simulink model "mpcmodel"  (R2023a)
settings: Solver=VariableStepAuto  StartTime=0.0  StopTime=21  RelTol=1e-3
undefined symbols (not defined in the file): C_aug, C_l, C_m, disc_sys, init, min_sampling_time, mpc_kalman_gain, P, potentiometer_linearity_percent, Q, V_bar, wave_amplitude, wave_period, x1_bar, x2_bar
libraries: mpclib x1
settings Model: Creator=yunzh  LastModifiedBy=yunzh

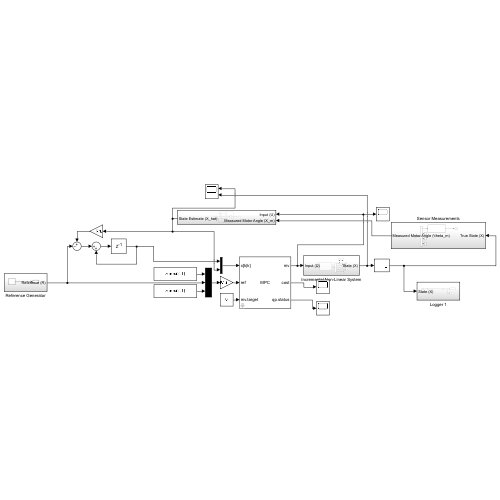
[thumbnail: Simulink's stored preview of the top-level diagram]
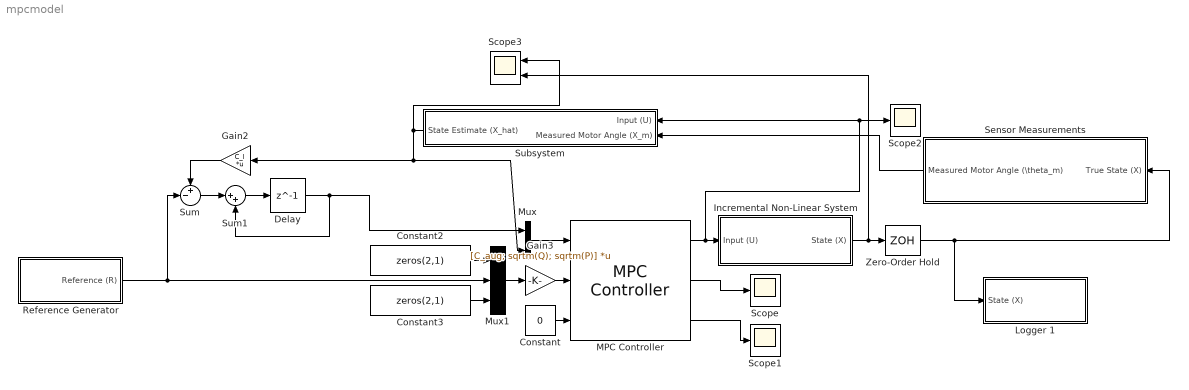
== system mpcmodel ==
  Constant : Constant  Value=0
  Constant2 : Constant  Value=zeros(2,1)
  Constant3 : Constant  Value=zeros(2,1)
  Delay : Delay  DelayLength=1  SampleTime=min_sampling_time
  Gain2 : Gain  Gain=C_l  Multiplication=Matrix(K*u)
  Gain3 : Gain  Gain=[C_aug; sqrtm(Q); sqrtm(P)]  Multiplication=Matrix(K*u)
  Incremental Non-Linear System : Subsystem
  Logger 1 : Subsystem
  MPC Controller : mpclib/MPC Controller  SCDEnableBlockLinearizationSpecification=on  mpcobj=mpc_obj  x0=mpc_initial_state  is_multiple=0  enable_value=0  return_u0=off  updateMPCinCallerWorkspace=on  md_inport=off  mv_inport=off  uref_inport=on  return_cost=on  return_mvseq=off  return_qpstatus=on  return_xseq=off  return_state=off  return_ovseq=off  state_inport=on  umin_inport=off  umax_inport=off  ymin_inport=off  ymax_inport=off  cc_inport=off  ywt_inport=off  uwt_inport=off  duwt_inport=off  rhoeps_inport=off  pm_inport=off  MaximumP=10  HorizonChoice=FixedHorizon  n_ts=0.02  n_p=20  n_mv=1  n_md=0  n_ud=0  n_mo=11  n_uo=0  BlockDataType=double  SampleTimeInherited=off  switch_inport=off
  Mux : Mux  Inputs=2
  Mux1 : Mux  Inputs=3
  Reference Generator : Subsystem
  Scope : Scope
  Scope1 : Scope
  Scope2 : Scope
  Scope3 : Scope  NumInputPorts=2
  Sensor Measurements : Subsystem
  Subsystem : Subsystem
  Sum : Sum  Inputs=+-|
  Sum1 : Sum  Inputs=|++
  Zero-Order Hold : ZeroOrderHold  SampleTime=min_sampling_time
  wires:
  Incremental Non-Linear System/1(State (X)) -> Scope3/2, Zero-Order Hold/1
  MPC Controller/1 -> Scope2/1, Subsystem/1(Input (U)), Incremental Non-Linear System/1(Input (U))
  Constant/1 -> MPC Controller/3
  Mux/1 -> MPC Controller/1
  Constant2/1 -> Mux1/1
  Reference Generator/1(Reference (R)) -> Mux1/2, Sum/2
  Constant3/1 -> Mux1/3
  Gain2/1 -> Sum/1
  Mux1/1 -> Gain3/1
  Gain3/1 -> MPC Controller/2
  MPC Controller/2 -> Scope/1
  MPC Controller/3 -> Scope1/1
  Sum/1 -> Sum1/1
  Sum1/1 -> Delay/1
  Zero-Order Hold/1 -> Sensor Measurements/1(True State (X)), Logger 1/1(State (X))
  Delay/1 -> Mux/1, Sum1/2
  Sensor Measurements/1(Measured Motor Angle (\theta_m)) -> Subsystem/2(Measured Motor Angle (X_m))
  Subsystem/1(State Estimate (X_hat)) -> Mux/2, Gain2/1, Scope3/1

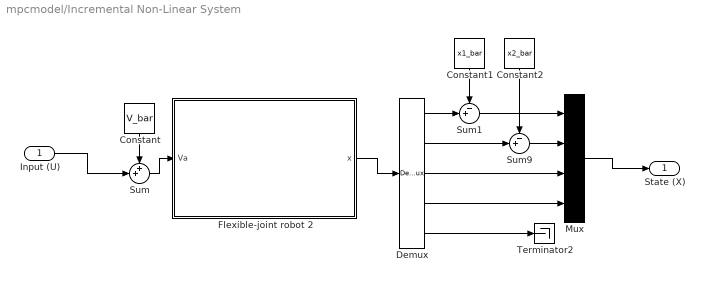
== system mpcmodel/Incremental Non-Linear System ==
  Input (U) : Inport
  Constant : Constant  Value=V_bar
  Constant1 : Constant  Value=x1_bar
  Constant2 : Constant  Value=x2_bar
  Demux : Demux  Outputs=5
  Flexible-joint robot 2 : Subsystem
      mask Display: image('$imagefile'); % Use "Edit Image" on toolstrip to change.
  Mux : Mux
  Sum : Sum  Inputs=++|
  Sum1 : Sum  Inputs=-+|
  Sum9 : Sum  Inputs=-+|
  Terminator2 : Terminator
  State (X) : Outport
  wires:
  Flexible-joint robot 2/1(x) -> Demux/1
  Demux/1 -> Sum1/2
  Demux/2 -> Sum9/2
  Demux/5 -> Terminator2/1
  Sum/1 -> Flexible-joint robot 2/1(Va)
  Constant1/1 -> Sum1/1
  Sum9/1 -> Mux/2
  Constant2/1 -> Sum9/1
  Sum1/1 -> Mux/1
  Demux/4 -> Mux/4
  Demux/3 -> Mux/3
  Constant/1 -> Sum/1
  Input (U)/1 -> Sum/2
  Mux/1 -> State (X)/1

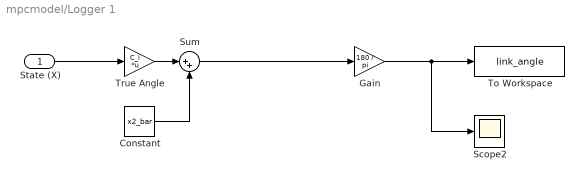
== system mpcmodel/Logger 1 ==
  State (X) : Inport
  Constant : Constant  Value=x2_bar
  Gain : Gain  Gain=180 / pi
  Scope2 : Scope
  Sum : Sum  Inputs=|++
  To Workspace : ToWorkspace  VariableName=link_angle  SaveFormat=Timeseries  SampleTime=-1
  True Angle : Gain  Gain=C_l  Multiplication=Matrix(K*u)
  wires:
  State (X)/1 -> True Angle/1
  True Angle/1 -> Sum/1
  Sum/1 -> Gain/1
  Gain/1 -> Scope2/1, To Workspace/1
  Constant/1 -> Sum/2

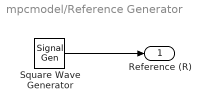
== system mpcmodel/Reference Generator ==
  Square Wave Generator : SignalGenerator  WaveForm=square  Amplitude=wave_amplitude  Frequency=1 / wave_period
  Reference (R) : Outport
  wires:
  Square Wave Generator/1 -> Reference (R)/1

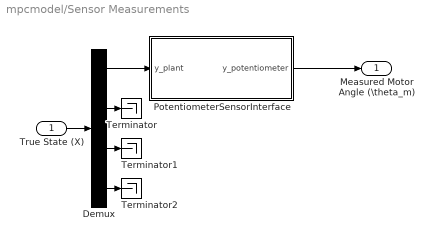
== system mpcmodel/Sensor Measurements ==
  True State (X) : Inport
  Demux : Demux
  PotentiometerSensorInterface : Subsystem  TreatAsAtomicUnit=on
      mask Display: image('$imagefile'); % Use "Edit Image" on toolstrip to change.
  Terminator : Terminator
  Terminator1 : Terminator
  Terminator2 : Terminator
  Measured Motor Angle (\theta_m) : Outport
  wires:
  Demux/1 -> PotentiometerSensorInterface/1(y_plant)
  True State (X)/1 -> Demux/1
  Demux/2 -> Terminator/1
  Demux/3 -> Terminator1/1
  Demux/4 -> Terminator2/1
  PotentiometerSensorInterface/1(y_potentiometer) -> Measured Motor Angle (\theta_m)/1

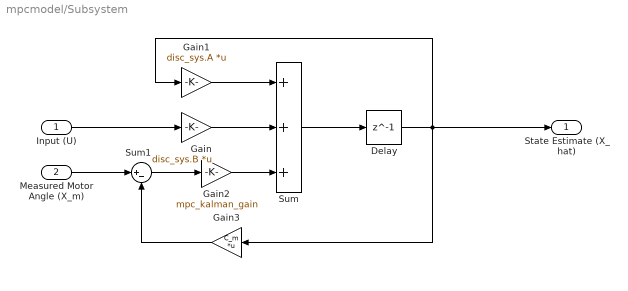
== system mpcmodel/Subsystem ==
  Input (U) : Inport
  Measured Motor Angle (X_m) : Inport  Port=2
  Delay : Delay  DelayLength=1  SampleTime=min_sampling_time
  Gain : Gain  Gain=disc_sys.B  Multiplication=Matrix(K*u)
  Gain1 : Gain  Gain=disc_sys.A  Multiplication=Matrix(K*u)
  Gain2 : Gain  Gain=mpc_kalman_gain
  Gain3 : Gain  Gain=C_m  Multiplication=Matrix(K*u)
  Sum : Sum  Inputs=+++
  Sum1 : Sum  Inputs=|+-
  State Estimate (X_hat) : Outport
  wires:
  Input (U)/1 -> Gain/1
  Gain/1 -> Sum/2
  Sum/1 -> Delay/1
  Delay/1 -> Gain3/1, Gain1/1, State Estimate (X_hat)/1
  Gain1/1 -> Sum/1
  Measured Motor Angle (X_m)/1 -> Sum1/1
  Sum1/1 -> Gain2/1
  Gain2/1 -> Sum/3
  Gain3/1 -> Sum1/2

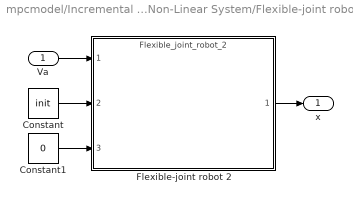
== system mpcmodel/Incremental Non-Linear System/Flexible-joint robot 2 ==
  Va : Inport
  Constant : Constant  Value=init
  Constant1 : Constant  Value=0
  Flexible-joint robot 2 : ModelReference  ModelNameDialog=Flexible_joint_robot_2  ModelReferenceVersion=1.65  CopyOfModelProtected=on
  x : Outport
  wires:
  Va/1 -> Flexible-joint robot 2/1
  Constant1/1 -> Flexible-joint robot 2/3
  Constant/1 -> Flexible-joint robot 2/2
  Flexible-joint robot 2/1 -> x/1

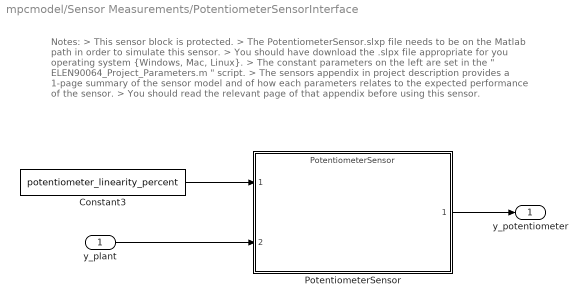
== system mpcmodel/Sensor Measurements/PotentiometerSensorInterface ==
  note: Notes:
      | > This sensor block is protected.
      | > The PotentiometerSensor.slxp file needs to be on the Matlab path in order to simulate this sensor.
      | > You should have download the .slpx file appropriate for you operating system {Windows, Mac, Linux}.
      | > The constant parameters on the left are set in the " ELEN90064_Project_Parameters.m " script.
      | > The sensors appendix in project description provides a 1-page summary of the sensor model and of how each parameters relates to the expected performance of the sensor.
      | > You should read the relevant page of that appendix before using this sensor.
  y_plant : Inport
  Constant3 : Constant  Value=potentiometer_linearity_percent
  PotentiometerSensor : ModelReference  ModelNameDialog=PotentiometerSensor.slxp  ModelReferenceVersion=1.21  CopyOfModelProtected=on
  y_potentiometer : Outport
  wires:
  y_plant/1 -> PotentiometerSensor/2
  Constant3/1 -> PotentiometerSensor/1
  PotentiometerSensor/1 -> y_potentiometer/1
